simulink model "model"  (R2020b)
settings: Solver=VariableStepAuto  StartTime=0.0  StopTime=100.0  MaxStep=0.001  RelTol=1e-3
settings Model: Creator=Vrunda M Balgi  LastModifiedBy=Vrunda M Balgi
settings DataIOCC: ExternalInput=[t, noise]  LoadExternalInput=on  SaveFormat=Array  SignalLogging=off  DSMLogging=off  ReturnWorkspaceOutputs=off

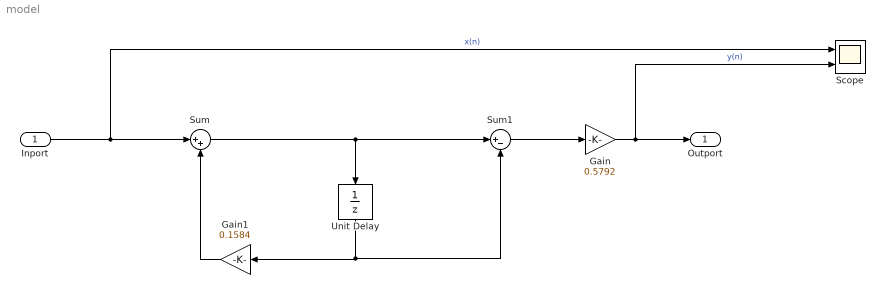
== system model ==
  Inport : Inport
  Gain : Gain  Gain=0.5792
  Gain1 : Gain  Gain=0.1584
  Scope : Scope  NumInputPorts=2
  Sum : Sum  Inputs=|++
  Sum1 : Sum  Inputs=|+-
  Unit Delay : UnitDelay  SampleTime=-1  HasFrameUpgradeWarning=on
  Outport : Outport
  wires:
  Sum/1 -> Unit Delay/1, Sum1/1
  Unit Delay/1 -> Sum1/2, Gain1/1
  Gain1/1 -> Sum/2
  Inport/1 -> Scope/1, Sum/1  "x(n)"
  Sum1/1 -> Gain/1
  Gain/1 -> Scope/2, Outport/1  "y(n)"
